simulink model "VCU_CS75_12_30_test"  (R2014a)
settings: Solver=FixedStepDiscrete  StartTime=0.0  StopTime=25  FixedStep=0.0005  RelTol=1e-3
InitFcn:
  | PID_canshu
values from neighbouring files (symbols this model uses):
  D1 = ecucoder_cal(D1)    [PID_canshu.m]
  D2 = ecucoder_cal(D2)    [PID_canshu.m]
  D3 = ecucoder_cal(D3)    [PID_canshu.m]
  ErrorLimit = ecucoder_cal(ErrorLimit)    [PID_canshu.m]
  ErrorSumMax1 = ecucoder_cal(ErrorSumMax1)    [PID_canshu.m]
  ErrorSumMax2 = ecucoder_cal(ErrorSumMax2)    [PID_canshu.m]
  ErrorSumMax3 = ecucoder_cal(ErrorSumMax3)    [PID_canshu.m]
  I1 = ecucoder_cal(I1)    [PID_canshu.m]
  I2 = ecucoder_cal(I2)    [PID_canshu.m]
  I3 = ecucoder_cal(I3)    [PID_canshu.m]
  Limit1 = ecucoder_cal(Limit1)    [PID_canshu.m]
  Limit2 = ecucoder_cal(Limit2)    [PID_canshu.m]
  P1 = ecucoder_cal(P1)    [PID_canshu.m]
  P2 = ecucoder_cal(P2)    [PID_canshu.m]
  P3 = ecucoder_cal(P3)    [PID_canshu.m]
  T_buchang = ecucoder_cal(T_buchang)    [PID_canshu.m]
undefined symbols (not defined in the file or in its folder): ecucoder_acal, I_SW01_L, LaterlAngleCommand, LDW, RemoteAcclPosition
libraries: simulink x940, ec5744lib x41
(part 19 of 31)

== system VCU_CS75_12_30_test/长安CS75底盘程序，20ms一次/Output/Subsystem/2E5/ACC_2E5/ACC_AEBLVehilcehold ==
  ACC_AEBLVehilcehold : Inport
  ACC_AEBLVehilceholdRon : Rounding  Operator=round
  ACC_AEBLVehilcehold_1sat : Saturate  UpperLimit=4  LowerLimit=0
  ACC_AEBLVehilcehold_Convert : DataTypeConversion  OutDataTypeStr=uint8
  ACC_AEBLVehilcehold_Convert1 : DataTypeConversion  OutDataTypeStr=uint32
  ACC_AEBLVehilcehold_D : Product  Inputs=*/
  ACC_AEBLVehilcehold_F : Constant  OutDataTypeStr=single
  ACC_AEBLVehilcehold_L : simulink/Logic and Bit Operations/Bitwise Operator  logicop=AND  UseBitMask=on  BitMask=4  BitMaskRealWorld=Stored Integer
  ACC_AEBLVehilcehold_O : Constant  Value=0  OutDataTypeStr=single
  ACC_AEBLVehilcehold_S : ArithShift  BitShiftNumber=-2
  ACC_AEBLVehilcehold_sat : Saturate  UpperLimit=1  LowerLimit=0
  ACC_AEBLVehilcehold_st : Sum  Inputs=+-
  Constant{1..3,5..8} (7 alike) : Constant  Value=0  OutDataTypeStr=uint8
  output1 : Outport
  output2 : Outport  Port=2
  output3 : Outport  Port=3
  output4 : Outport  Port=4
  output5 : Outport  Port=5
  output6 : Outport  Port=6
  output7 : Outport  Port=7
  output8 : Outport  Port=8
  wires:
  ACC_AEBLVehilcehold/1 -> ACC_AEBLVehilcehold_sat/1
  ACC_AEBLVehilcehold_sat/1 -> ACC_AEBLVehilcehold_st/1
  ACC_AEBLVehilcehold_O/1 -> ACC_AEBLVehilcehold_st/2
  ACC_AEBLVehilcehold_st/1 -> ACC_AEBLVehilcehold_D/1
  ACC_AEBLVehilcehold_F/1 -> ACC_AEBLVehilcehold_D/2
  ACC_AEBLVehilcehold_D/1 -> ACC_AEBLVehilceholdRon/1
  ACC_AEBLVehilceholdRon/1 -> ACC_AEBLVehilcehold_S/1
  ACC_AEBLVehilcehold_S/1 -> ACC_AEBLVehilcehold_1sat/1
  ACC_AEBLVehilcehold_1sat/1 -> ACC_AEBLVehilcehold_Convert1/1
  ACC_AEBLVehilcehold_Convert1/1 -> ACC_AEBLVehilcehold_L/1
  ACC_AEBLVehilcehold_L/1 -> ACC_AEBLVehilcehold_Convert/1
  ACC_AEBLVehilcehold_Convert/1 -> output4/1
  Constant1/1 -> output1/1
  Constant2/1 -> output2/1
  Constant3/1 -> output3/1
  Constant5/1 -> output5/1
  Constant6/1 -> output6/1
  Constant7/1 -> output7/1
  Constant8/1 -> output8/1

== system VCU_CS75_12_30_test/长安CS75底盘程序，20ms一次/Output/Subsystem/2E5/ACC_2E5/ACC_AEBTargetDeceleration ==
  ACC_AEBTargetDeceleration : Inport
  ACC_AEBTargetDecelerationBitCov : DataTypeConversion  OutDataTypeStr=uint32
  ACC_AEBTargetDecelerationBitCov1 : DataTypeConversion  OutDataTypeStr=uint8
  ACC_AEBTargetDecelerationCOV : DataTypeConversion  OutDataTypeStr=uint8
  ACC_AEBTargetDecelerationCOV1 : DataTypeConversion  OutDataTypeStr=uint8
  ACC_AEBTargetDecelerationRon : Rounding  Operator=round
  ACC_AEBTargetDeceleration_1sat : Saturate  UpperLimit=2097120  LowerLimit=0
  ACC_AEBTargetDeceleration_And : simulink/Logic and Bit Operations/Bitwise Operator  logicop=AND  UseBitMask=off  NumInputPorts=2  BitMask=bin2dec('11011001')  BitMaskRealWorld=Stored Integer
  ACC_AEBTargetDeceleration_And1 : simulink/Logic and Bit Operations/Bitwise Operator  logicop=AND  UseBitMask=off  NumInputPorts=2  BitMask=bin2dec('11011001')  BitMaskRealWorld=Stored Integer
  ACC_AEBTargetDeceleration_And1_C : Constant  Value=255  OutDataTypeStr=uint32
  ACC_AEBTargetDeceleration_And_C : Constant  Value=65535
  ACC_AEBTargetDeceleration_Convert : DataTypeConversion  OutDataTypeStr=uint32
  ACC_AEBTargetDeceleration_D : Product  Inputs=*/
  ACC_AEBTargetDeceleration_D1 : Product  Inputs=*/
  ACC_AEBTargetDeceleration_D2 : Product  Inputs=*/
  ACC_AEBTargetDeceleration_F : Constant  Value=0.0005  OutDataTypeStr=single
  ACC_AEBTargetDeceleration_L : simulink/Logic and Bit Operations/Bitwise Operator  logicop=AND  UseBitMask=on  BitMask=2097120  BitMaskRealWorld=Stored Integer
  ACC_AEBTargetDeceleration_O : Constant  Value=-16  OutDataTypeStr=single
  ACC_AEBTargetDeceleration_S : ArithShift  BitShiftNumber=-5
  ACC_AEBTargetDeceleration_sat : Saturate  UpperLimit=16  LowerLimit=-16
  ACC_AEBTargetDeceleration_st : Sum  Inputs=+-
  ACC_AEBTargetDecelerationoutput1_C : Constant  Value=65536
  ACC_AEBTargetDecelerationoutput2_C : Constant  Value=256
  Constant{4..8} (5 alike) : Constant  Value=0  OutDataTypeStr=uint8
  output1 : Outport
  output2 : Outport  Port=2
  output3 : Outport  Port=3
  output4 : Outport  Port=4
  output5 : Outport  Port=5
  output6 : Outport  Port=6
  output7 : Outport  Port=7
  output8 : Outport  Port=8
  wires:
  ACC_AEBTargetDeceleration/1 -> ACC_AEBTargetDeceleration_sat/1
  ACC_AEBTargetDeceleration_sat/1 -> ACC_AEBTargetDeceleration_st/1
  ACC_AEBTargetDeceleration_O/1 -> ACC_AEBTargetDeceleration_st/2
  ACC_AEBTargetDeceleration_st/1 -> ACC_AEBTargetDeceleration_D/1
  ACC_AEBTargetDeceleration_F/1 -> ACC_AEBTargetDeceleration_D/2
  ACC_AEBTargetDeceleration_D/1 -> ACC_AEBTargetDecelerationRon/1
  ACC_AEBTargetDecelerationRon/1 -> ACC_AEBTargetDeceleration_S/1
  ACC_AEBTargetDeceleration_S/1 -> ACC_AEBTargetDeceleration_1sat/1
  ACC_AEBTargetDeceleration_1sat/1 -> ACC_AEBTargetDeceleration_Convert/1
  ACC_AEBTargetDeceleration_Convert/1 -> ACC_AEBTargetDeceleration_L/1
  ACC_AEBTargetDeceleration_L/1 -> ACC_AEBTargetDeceleration_D1/1, ACC_AEBTargetDeceleration_And/1, ACC_AEBTargetDeceleration_And1/1
  ACC_AEBTargetDecelerationoutput1_C/1 -> ACC_AEBTargetDeceleration_D1/2
  ACC_AEBTargetDeceleration_D1/1 -> ACC_AEBTargetDecelerationCOV/1
  ACC_AEBTargetDecelerationCOV/1 -> output1/1
  ACC_AEBTargetDeceleration_And_C/1 -> ACC_AEBTargetDecelerationBitCov/1
  ACC_AEBTargetDecelerationBitCov/1 -> ACC_AEBTargetDeceleration_And/2
  ACC_AEBTargetDeceleration_And/1 -> ACC_AEBTargetDeceleration_D2/1
  ACC_AEBTargetDecelerationoutput2_C/1 -> ACC_AEBTargetDeceleration_D2/2
  ACC_AEBTargetDeceleration_D2/1 -> ACC_AEBTargetDecelerationCOV1/1
  ACC_AEBTargetDecelerationCOV1/1 -> output2/1
  ACC_AEBTargetDeceleration_And1_C/1 -> ACC_AEBTargetDeceleration_And1/2
  ACC_AEBTargetDeceleration_And1/1 -> ACC_AEBTargetDecelerationBitCov1/1
  ACC_AEBTargetDecelerationBitCov1/1 -> output3/1
  Constant4/1 -> output4/1
  Constant5/1 -> output5/1
  Constant6/1 -> output6/1
  Constant7/1 -> output7/1
  Constant8/1 -> output8/1

== system VCU_CS75_12_30_test/长安CS75底盘程序，20ms一次/Output/Subsystem/2E5/ACC_2E5/ACC_AWBavailable ==
  ACC_AWBavailable : Inport
  ACC_AWBavailableRon : Rounding  Operator=round
  ACC_AWBavailable_1sat : Saturate  UpperLimit=128  LowerLimit=0
  ACC_AWBavailable_Convert : DataTypeConversion  OutDataTypeStr=uint8
  ACC_AWBavailable_Convert1 : DataTypeConversion  OutDataTypeStr=uint32
  ACC_AWBavailable_D : Product  Inputs=*/
  ACC_AWBavailable_F : Constant  OutDataTypeStr=single
  ACC_AWBavailable_L : simulink/Logic and Bit Operations/Bitwise Operator  logicop=AND  UseBitMask=on  BitMask=128  BitMaskRealWorld=Stored Integer
  ACC_AWBavailable_O : Constant  Value=0  OutDataTypeStr=single
  ACC_AWBavailable_S : ArithShift  BitShiftNumber=-7
  ACC_AWBavailable_sat : Saturate  UpperLimit=1  LowerLimit=0
  ACC_AWBavailable_st : Sum  Inputs=+-
  Constant{1..3,5..8} (7 alike) : Constant  Value=0  OutDataTypeStr=uint8
  output1 : Outport
  output2 : Outport  Port=2
  output3 : Outport  Port=3
  output4 : Outport  Port=4
  output5 : Outport  Port=5
  output6 : Outport  Port=6
  output7 : Outport  Port=7
  output8 : Outport  Port=8
  wires:
  ACC_AWBavailable/1 -> ACC_AWBavailable_sat/1
  ACC_AWBavailable_sat/1 -> ACC_AWBavailable_st/1
  ACC_AWBavailable_O/1 -> ACC_AWBavailable_st/2
  ACC_AWBavailable_st/1 -> ACC_AWBavailable_D/1
  ACC_AWBavailable_F/1 -> ACC_AWBavailable_D/2
  ACC_AWBavailable_D/1 -> ACC_AWBavailableRon/1
  ACC_AWBavailableRon/1 -> ACC_AWBavailable_S/1
  ACC_AWBavailable_S/1 -> ACC_AWBavailable_1sat/1
  ACC_AWBavailable_1sat/1 -> ACC_AWBavailable_Convert1/1
  ACC_AWBavailable_Convert1/1 -> ACC_AWBavailable_L/1
  ACC_AWBavailable_L/1 -> ACC_AWBavailable_Convert/1
  ACC_AWBavailable_Convert/1 -> output4/1
  Constant1/1 -> output1/1
  Constant2/1 -> output2/1
  Constant3/1 -> output3/1
  Constant5/1 -> output5/1
  Constant6/1 -> output6/1
  Constant7/1 -> output7/1
  Constant8/1 -> output8/1

== system VCU_CS75_12_30_test/长安CS75底盘程序，20ms一次/Output/Subsystem/2E5/ACC_2E5/ACC_AWBlevel ==
  ACC_AWBlevel : Inport
  ACC_AWBlevelRon : Rounding  Operator=round
  ACC_AWBlevel_1sat : Saturate  UpperLimit=15  LowerLimit=0
  ACC_AWBlevel_Convert : DataTypeConversion  OutDataTypeStr=uint8
  ACC_AWBlevel_Convert1 : DataTypeConversion  OutDataTypeStr=uint32
  ACC_AWBlevel_D : Product  Inputs=*/
  ACC_AWBlevel_F : Constant  OutDataTypeStr=single
  ACC_AWBlevel_L : simulink/Logic and Bit Operations/Bitwise Operator  logicop=AND  UseBitMask=on  BitMask=15  BitMaskRealWorld=Stored Integer
  ACC_AWBlevel_O : Constant  Value=0  OutDataTypeStr=single
  ACC_AWBlevel_S : ArithShift
  ACC_AWBlevel_sat : Saturate  UpperLimit=15  LowerLimit=0
  ACC_AWBlevel_st : Sum  Inputs=+-
  Constant{1..2,4..8} (7 alike) : Constant  Value=0  OutDataTypeStr=uint8
  output1 : Outport
  output2 : Outport  Port=2
  output3 : Outport  Port=3
  output4 : Outport  Port=4
  output5 : Outport  Port=5
  output6 : Outport  Port=6
  output7 : Outport  Port=7
  output8 : Outport  Port=8
  wires:
  ACC_AWBlevel/1 -> ACC_AWBlevel_sat/1
  ACC_AWBlevel_sat/1 -> ACC_AWBlevel_st/1
  ACC_AWBlevel_O/1 -> ACC_AWBlevel_st/2
  ACC_AWBlevel_st/1 -> ACC_AWBlevel_D/1
  ACC_AWBlevel_F/1 -> ACC_AWBlevel_D/2
  ACC_AWBlevel_D/1 -> ACC_AWBlevelRon/1
  ACC_AWBlevelRon/1 -> ACC_AWBlevel_S/1
  ACC_AWBlevel_S/1 -> ACC_AWBlevel_1sat/1
  ACC_AWBlevel_1sat/1 -> ACC_AWBlevel_Convert1/1
  ACC_AWBlevel_Convert1/1 -> ACC_AWBlevel_L/1
  ACC_AWBlevel_L/1 -> ACC_AWBlevel_Convert/1
  ACC_AWBlevel_Convert/1 -> output3/1
  Constant1/1 -> output1/1
  Constant2/1 -> output2/1
  Constant4/1 -> output4/1
  Constant5/1 -> output5/1
  Constant6/1 -> output6/1
  Constant7/1 -> output7/1
  Constant8/1 -> output8/1

== system VCU_CS75_12_30_test/长安CS75底盘程序，20ms一次/Output/Subsystem/2E5/ACC_2E5/ACC_AccTorqueReq ==
  ACC_AccTorqueReq : Inport
  ACC_AccTorqueReqBitCov : DataTypeConversion  OutDataTypeStr=uint8
  ACC_AccTorqueReqCOV : DataTypeConversion  OutDataTypeStr=uint8
  ACC_AccTorqueReqRon : Rounding  Operator=round
  ACC_AccTorqueReq_1sat : Saturate  UpperLimit=4092  LowerLimit=0
  ACC_AccTorqueReq_And : simulink/Logic and Bit Operations/Bitwise Operator  logicop=AND  UseBitMask=off  NumInputPorts=2  BitMask=bin2dec('11011001')  BitMaskRealWorld=Stored Integer
  ACC_AccTorqueReq_And_C : Constant  Value=255  OutDataTypeStr=uint32
  ACC_AccTorqueReq_Convert : DataTypeConversion  OutDataTypeStr=uint32
  ACC_AccTorqueReq_D : Product  Inputs=*/
  ACC_AccTorqueReq_D1 : Product  Inputs=*/
  ACC_AccTorqueReq_F : Constant  Value=0.09784  OutDataTypeStr=single
  ACC_AccTorqueReq_L : simulink/Logic and Bit Operations/Bitwise Operator  logicop=AND  UseBitMask=on  BitMask=4092  BitMaskRealWorld=Stored Integer
  ACC_AccTorqueReq_O : Constant  Value=0  OutDataTypeStr=single
  ACC_AccTorqueReq_S : ArithShift  BitShiftNumber=-2
  ACC_AccTorqueReq_sat : Saturate  UpperLimit=100.09032  LowerLimit=0
  ACC_AccTorqueReq_st : Sum  Inputs=+-
  ACC_AccTorqueReqoutput5_C : Constant  Value=256
  Constant{1..4,7..8} (6 alike) : Constant  Value=0  OutDataTypeStr=uint8
  output1 : Outport
  output2 : Outport  Port=2
  output3 : Outport  Port=3
  output4 : Outport  Port=4
  output5 : Outport  Port=5
  output6 : Outport  Port=6
  output7 : Outport  Port=7
  output8 : Outport  Port=8
  wires:
  ACC_AccTorqueReq/1 -> ACC_AccTorqueReq_sat/1
  ACC_AccTorqueReq_sat/1 -> ACC_AccTorqueReq_st/1
  ACC_AccTorqueReq_O/1 -> ACC_AccTorqueReq_st/2
  ACC_AccTorqueReq_st/1 -> ACC_AccTorqueReq_D/1
  ACC_AccTorqueReq_F/1 -> ACC_AccTorqueReq_D/2
  ACC_AccTorqueReq_D/1 -> ACC_AccTorqueReqRon/1
  ACC_AccTorqueReqRon/1 -> ACC_AccTorqueReq_S/1
  ACC_AccTorqueReq_S/1 -> ACC_AccTorqueReq_1sat/1
  ACC_AccTorqueReq_1sat/1 -> ACC_AccTorqueReq_Convert/1
  ACC_AccTorqueReq_Convert/1 -> ACC_AccTorqueReq_L/1
  ACC_AccTorqueReq_L/1 -> ACC_AccTorqueReq_D1/1, ACC_AccTorqueReq_And/1
  ACC_AccTorqueReqoutput5_C/1 -> ACC_AccTorqueReq_D1/2
  ACC_AccTorqueReq_D1/1 -> ACC_AccTorqueReqCOV/1
  ACC_AccTorqueReqCOV/1 -> output5/1
  ACC_AccTorqueReq_And_C/1 -> ACC_AccTorqueReq_And/2
  ACC_AccTorqueReq_And/1 -> ACC_AccTorqueReqBitCov/1
  ACC_AccTorqueReqBitCov/1 -> output6/1
  Constant1/1 -> output1/1
  Constant2/1 -> output2/1
  Constant3/1 -> output3/1
  Constant4/1 -> output4/1
  Constant7/1 -> output7/1
  Constant8/1 -> output8/1

== system VCU_CS75_12_30_test/长安CS75底盘程序，20ms一次/Output/Subsystem/2E5/ACC_2E5/ACC_AccTrqReqEnable ==
  ACC_AccTrqReqEnable : Inport
  ACC_AccTrqReqEnableRon : Rounding  Operator=round
  ACC_AccTrqReqEnable_1sat : Saturate  UpperLimit=128  LowerLimit=0
  ACC_AccTrqReqEnable_Convert : DataTypeConversion  OutDataTypeStr=uint8
  ACC_AccTrqReqEnable_Convert1 : DataTypeConversion  OutDataTypeStr=uint32
  ACC_AccTrqReqEnable_D : Product  Inputs=*/
  ACC_AccTrqReqEnable_F : Constant  OutDataTypeStr=single
  ACC_AccTrqReqEnable_L : simulink/Logic and Bit Operations/Bitwise Operator  logicop=AND  UseBitMask=on  BitMask=128  BitMaskRealWorld=Stored Integer
  ACC_AccTrqReqEnable_O : Constant  Value=0  OutDataTypeStr=single
  ACC_AccTrqReqEnable_S : ArithShift  BitShiftNumber=-7
  ACC_AccTrqReqEnable_sat : Saturate  UpperLimit=1  LowerLimit=0
  ACC_AccTrqReqEnable_st : Sum  Inputs=+-
  Constant{2..8} (7 alike) : Constant  Value=0  OutDataTypeStr=uint8
  output1 : Outport
  output2 : Outport  Port=2
  output3 : Outport  Port=3
  output4 : Outport  Port=4
  output5 : Outport  Port=5
  output6 : Outport  Port=6
  output7 : Outport  Port=7
  output8 : Outport  Port=8
  wires:
  ACC_AccTrqReqEnable/1 -> ACC_AccTrqReqEnable_sat/1
  ACC_AccTrqReqEnable_sat/1 -> ACC_AccTrqReqEnable_st/1
  ACC_AccTrqReqEnable_O/1 -> ACC_AccTrqReqEnable_st/2
  ACC_AccTrqReqEnable_st/1 -> ACC_AccTrqReqEnable_D/1
  ACC_AccTrqReqEnable_F/1 -> ACC_AccTrqReqEnable_D/2
  ACC_AccTrqReqEnable_D/1 -> ACC_AccTrqReqEnableRon/1
  ACC_AccTrqReqEnableRon/1 -> ACC_AccTrqReqEnable_S/1
  ACC_AccTrqReqEnable_S/1 -> ACC_AccTrqReqEnable_1sat/1
  ACC_AccTrqReqEnable_1sat/1 -> ACC_AccTrqReqEnable_Convert1/1
  ACC_AccTrqReqEnable_Convert1/1 -> ACC_AccTrqReqEnable_L/1
  ACC_AccTrqReqEnable_L/1 -> ACC_AccTrqReqEnable_Convert/1
  ACC_AccTrqReqEnable_Convert/1 -> output1/1
  Constant2/1 -> output2/1
  Constant3/1 -> output3/1
  Constant4/1 -> output4/1
  Constant5/1 -> output5/1
  Constant6/1 -> output6/1
  Constant7/1 -> output7/1
  Constant8/1 -> output8/1

== system VCU_CS75_12_30_test/长安CS75底盘程序，20ms一次/Output/Subsystem/2E5/ACC_2E5/ACC_CheckSum ==
  ACC_CheckSum : Inport
  ACC_CheckSumRon : Rounding  Operator=round
  ACC_CheckSum_1sat : Saturate  UpperLimit=255  LowerLimit=0
  ACC_CheckSum_Convert : DataTypeConversion  OutDataTypeStr=uint8
  ACC_CheckSum_Convert1 : DataTypeConversion  OutDataTypeStr=uint32
  ACC_CheckSum_D : Product  Inputs=*/
  ACC_CheckSum_F : Constant  OutDataTypeStr=single
  ACC_CheckSum_L : simulink/Logic and Bit Operations/Bitwise Operator  logicop=AND  UseBitMask=on  BitMask=255  BitMaskRealWorld=Stored Integer
  ACC_CheckSum_O : Constant  Value=0  OutDataTypeStr=single
  ACC_CheckSum_S : ArithShift
  ACC_CheckSum_sat : Saturate  UpperLimit=255  LowerLimit=0
  ACC_CheckSum_st : Sum  Inputs=+-
  Constant{1..7} (7 alike) : Constant  Value=0  OutDataTypeStr=uint8
  output1 : Outport
  output2 : Outport  Port=2
  output3 : Outport  Port=3
  output4 : Outport  Port=4
  output5 : Outport  Port=5
  output6 : Outport  Port=6
  output7 : Outport  Port=7
  output8 : Outport  Port=8
  wires:
  ACC_CheckSum/1 -> ACC_CheckSum_sat/1
  ACC_CheckSum_sat/1 -> ACC_CheckSum_st/1
  ACC_CheckSum_O/1 -> ACC_CheckSum_st/2
  ACC_CheckSum_st/1 -> ACC_CheckSum_D/1
  ACC_CheckSum_F/1 -> ACC_CheckSum_D/2
  ACC_CheckSum_D/1 -> ACC_CheckSumRon/1
  ACC_CheckSumRon/1 -> ACC_CheckSum_S/1
  ACC_CheckSum_S/1 -> ACC_CheckSum_1sat/1
  ACC_CheckSum_1sat/1 -> ACC_CheckSum_Convert1/1
  ACC_CheckSum_Convert1/1 -> ACC_CheckSum_L/1
  ACC_CheckSum_L/1 -> ACC_CheckSum_Convert/1
  ACC_CheckSum_Convert/1 -> output8/1
  Constant1/1 -> output1/1
  Constant2/1 -> output2/1
  Constant3/1 -> output3/1
  Constant4/1 -> output4/1
  Constant5/1 -> output5/1
  Constant6/1 -> output6/1
  Constant7/1 -> output7/1

== system VCU_CS75_12_30_test/长安CS75底盘程序，20ms一次/Output/Subsystem/2E5/ACC_2E5/ACC_ESPPrefill ==
  ACC_ESPPrefill : Inport
  ACC_ESPPrefillRon : Rounding  Operator=round
  ACC_ESPPrefill_1sat : Saturate  UpperLimit=64  LowerLimit=0
  ACC_ESPPrefill_Convert : DataTypeConversion  OutDataTypeStr=uint8
  ACC_ESPPrefill_Convert1 : DataTypeConversion  OutDataTypeStr=uint32
  ACC_ESPPrefill_D : Product  Inputs=*/
  ACC_ESPPrefill_F : Constant  OutDataTypeStr=single
  ACC_ESPPrefill_L : simulink/Logic and Bit Operations/Bitwise Operator  logicop=AND  UseBitMask=on  BitMask=64  BitMaskRealWorld=Stored Integer
  ACC_ESPPrefill_O : Constant  Value=0  OutDataTypeStr=single
  ACC_ESPPrefill_S : ArithShift  BitShiftNumber=-6
  ACC_ESPPrefill_sat : Saturate  UpperLimit=1  LowerLimit=0
  ACC_ESPPrefill_st : Sum  Inputs=+-
  Constant{1..3,5..8} (7 alike) : Constant  Value=0  OutDataTypeStr=uint8
  output1 : Outport
  output2 : Outport  Port=2
  output3 : Outport  Port=3
  output4 : Outport  Port=4
  output5 : Outport  Port=5
  output6 : Outport  Port=6
  output7 : Outport  Port=7
  output8 : Outport  Port=8
  wires:
  ACC_ESPPrefill/1 -> ACC_ESPPrefill_sat/1
  ACC_ESPPrefill_sat/1 -> ACC_ESPPrefill_st/1
  ACC_ESPPrefill_O/1 -> ACC_ESPPrefill_st/2
  ACC_ESPPrefill_st/1 -> ACC_ESPPrefill_D/1
  ACC_ESPPrefill_F/1 -> ACC_ESPPrefill_D/2
  ACC_ESPPrefill_D/1 -> ACC_ESPPrefillRon/1
  ACC_ESPPrefillRon/1 -> ACC_ESPPrefill_S/1
  ACC_ESPPrefill_S/1 -> ACC_ESPPrefill_1sat/1
  ACC_ESPPrefill_1sat/1 -> ACC_ESPPrefill_Convert1/1
  ACC_ESPPrefill_Convert1/1 -> ACC_ESPPrefill_L/1
  ACC_ESPPrefill_L/1 -> ACC_ESPPrefill_Convert/1
  ACC_ESPPrefill_Convert/1 -> output4/1
  Constant1/1 -> output1/1
  Constant2/1 -> output2/1
  Constant3/1 -> output3/1
  Constant5/1 -> output5/1
  Constant6/1 -> output6/1
  Constant7/1 -> output7/1
  Constant8/1 -> output8/1

== system VCU_CS75_12_30_test/长安CS75底盘程序，20ms一次/Output/Subsystem/2E5/ACC_2E5/ACC_PCWPenable ==
  ACC_PCWPenable : Inport
  ACC_PCWPenableRon : Rounding  Operator=round
  ACC_PCWPenable_1sat : Saturate  UpperLimit=32  LowerLimit=0
  ACC_PCWPenable_Convert : DataTypeConversion  OutDataTypeStr=uint8
  ACC_PCWPenable_Convert1 : DataTypeConversion  OutDataTypeStr=uint32
  ACC_PCWPenable_D : Product  Inputs=*/
  ACC_PCWPenable_F : Constant  OutDataTypeStr=single
  ACC_PCWPenable_L : simulink/Logic and Bit Operations/Bitwise Operator  logicop=AND  UseBitMask=on  BitMask=32  BitMaskRealWorld=Stored Integer
  ACC_PCWPenable_O : Constant  Value=0  OutDataTypeStr=single
  ACC_PCWPenable_S : ArithShift  BitShiftNumber=-5
  ACC_PCWPenable_sat : Saturate  UpperLimit=1  LowerLimit=0
  ACC_PCWPenable_st : Sum  Inputs=+-
  Constant{1..3,5..8} (7 alike) : Constant  Value=0  OutDataTypeStr=uint8
  output1 : Outport
  output2 : Outport  Port=2
  output3 : Outport  Port=3
  output4 : Outport  Port=4
  output5 : Outport  Port=5
  output6 : Outport  Port=6
  output7 : Outport  Port=7
  output8 : Outport  Port=8
  wires:
  ACC_PCWPenable/1 -> ACC_PCWPenable_sat/1
  ACC_PCWPenable_sat/1 -> ACC_PCWPenable_st/1
  ACC_PCWPenable_O/1 -> ACC_PCWPenable_st/2
  ACC_PCWPenable_st/1 -> ACC_PCWPenable_D/1
  ACC_PCWPenable_F/1 -> ACC_PCWPenable_D/2
  ACC_PCWPenable_D/1 -> ACC_PCWPenableRon/1
  ACC_PCWPenableRon/1 -> ACC_PCWPenable_S/1
  ACC_PCWPenable_S/1 -> ACC_PCWPenable_1sat/1
  ACC_PCWPenable_1sat/1 -> ACC_PCWPenable_Convert1/1
  ACC_PCWPenable_Convert1/1 -> ACC_PCWPenable_L/1
  ACC_PCWPenable_L/1 -> ACC_PCWPenable_Convert/1
  ACC_PCWPenable_Convert/1 -> output4/1
  Constant1/1 -> output1/1
  Constant2/1 -> output2/1
  Constant3/1 -> output3/1
  Constant5/1 -> output5/1
  Constant6/1 -> output6/1
  Constant7/1 -> output7/1
  Constant8/1 -> output8/1

== system VCU_CS75_12_30_test/长安CS75底盘程序，20ms一次/Output/Subsystem/2E5/ACC_2E5/ACC_PCWPreWarning ==
  ACC_PCWPreWarning : Inport
  ACC_PCWPreWarningRon : Rounding  Operator=round
  ACC_PCWPreWarning_1sat : Saturate  UpperLimit=8  LowerLimit=0
  ACC_PCWPreWarning_Convert : DataTypeConversion  OutDataTypeStr=uint8
  ACC_PCWPreWarning_Convert1 : DataTypeConversion  OutDataTypeStr=uint32
  ACC_PCWPreWarning_D : Product  Inputs=*/
  ACC_PCWPreWarning_F : Constant  OutDataTypeStr=single
  ACC_PCWPreWarning_L : simulink/Logic and Bit Operations/Bitwise Operator  logicop=AND  UseBitMask=on  BitMask=8  BitMaskRealWorld=Stored Integer
  ACC_PCWPreWarning_O : Constant  Value=0  OutDataTypeStr=single
  ACC_PCWPreWarning_S : ArithShift  BitShiftNumber=-3
  ACC_PCWPreWarning_sat : Saturate  UpperLimit=0  LowerLimit=0
  ACC_PCWPreWarning_st : Sum  Inputs=+-
  Constant{1..3,5..8} (7 alike) : Constant  Value=0  OutDataTypeStr=uint8
  output1 : Outport
  output2 : Outport  Port=2
  output3 : Outport  Port=3
  output4 : Outport  Port=4
  output5 : Outport  Port=5
  output6 : Outport  Port=6
  output7 : Outport  Port=7
  output8 : Outport  Port=8
  wires:
  ACC_PCWPreWarning/1 -> ACC_PCWPreWarning_sat/1
  ACC_PCWPreWarning_sat/1 -> ACC_PCWPreWarning_st/1
  ACC_PCWPreWarning_O/1 -> ACC_PCWPreWarning_st/2
  ACC_PCWPreWarning_st/1 -> ACC_PCWPreWarning_D/1
  ACC_PCWPreWarning_F/1 -> ACC_PCWPreWarning_D/2
  ACC_PCWPreWarning_D/1 -> ACC_PCWPreWarningRon/1
  ACC_PCWPreWarningRon/1 -> ACC_PCWPreWarning_S/1
  ACC_PCWPreWarning_S/1 -> ACC_PCWPreWarning_1sat/1
  ACC_PCWPreWarning_1sat/1 -> ACC_PCWPreWarning_Convert1/1
  ACC_PCWPreWarning_Convert1/1 -> ACC_PCWPreWarning_L/1
  ACC_PCWPreWarning_L/1 -> ACC_PCWPreWarning_Convert/1
  ACC_PCWPreWarning_Convert/1 -> output4/1
  Constant1/1 -> output1/1
  Constant2/1 -> output2/1
  Constant3/1 -> output3/1
  Constant5/1 -> output5/1
  Constant6/1 -> output6/1
  Constant7/1 -> output7/1
  Constant8/1 -> output8/1

== system VCU_CS75_12_30_test/长安CS75底盘程序，20ms一次/Output/Subsystem/2E5/ACC_2E5/ACC_PCW_LatentWarning ==
  ACC_PCW_LatentWarning : Inport
  ACC_PCW_LatentWarningRon : Rounding  Operator=round
  ACC_PCW_LatentWarning_1sat : Saturate  UpperLimit=16  LowerLimit=0
  ACC_PCW_LatentWarning_Convert : DataTypeConversion  OutDataTypeStr=uint8
  ACC_PCW_LatentWarning_Convert1 : DataTypeConversion  OutDataTypeStr=uint32
  ACC_PCW_LatentWarning_D : Product  Inputs=*/
  ACC_PCW_LatentWarning_F : Constant  OutDataTypeStr=single
  ACC_PCW_LatentWarning_L : simulink/Logic and Bit Operations/Bitwise Operator  logicop=AND  UseBitMask=on  BitMask=16  BitMaskRealWorld=Stored Integer
  ACC_PCW_LatentWarning_O : Constant  Value=0  OutDataTypeStr=single
  ACC_PCW_LatentWarning_S : ArithShift  BitShiftNumber=-4
  ACC_PCW_LatentWarning_sat : Saturate  UpperLimit=0  LowerLimit=0
  ACC_PCW_LatentWarning_st : Sum  Inputs=+-
  Constant{1..3,5..8} (7 alike) : Constant  Value=0  OutDataTypeStr=uint8
  output1 : Outport
  output2 : Outport  Port=2
  output3 : Outport  Port=3
  output4 : Outport  Port=4
  output5 : Outport  Port=5
  output6 : Outport  Port=6
  output7 : Outport  Port=7
  output8 : Outport  Port=8
  wires:
  ACC_PCW_LatentWarning/1 -> ACC_PCW_LatentWarning_sat/1
  ACC_PCW_LatentWarning_sat/1 -> ACC_PCW_LatentWarning_st/1
  ACC_PCW_LatentWarning_O/1 -> ACC_PCW_LatentWarning_st/2
  ACC_PCW_LatentWarning_st/1 -> ACC_PCW_LatentWarning_D/1
  ACC_PCW_LatentWarning_F/1 -> ACC_PCW_LatentWarning_D/2
  ACC_PCW_LatentWarning_D/1 -> ACC_PCW_LatentWarningRon/1
  ACC_PCW_LatentWarningRon/1 -> ACC_PCW_LatentWarning_S/1
  ACC_PCW_LatentWarning_S/1 -> ACC_PCW_LatentWarning_1sat/1
  ACC_PCW_LatentWarning_1sat/1 -> ACC_PCW_LatentWarning_Convert1/1
  ACC_PCW_LatentWarning_Convert1/1 -> ACC_PCW_LatentWarning_L/1
  ACC_PCW_LatentWarning_L/1 -> ACC_PCW_LatentWarning_Convert/1
  ACC_PCW_LatentWarning_Convert/1 -> output4/1
  Constant1/1 -> output1/1
  Constant2/1 -> output2/1
  Constant3/1 -> output3/1
  Constant5/1 -> output5/1
  Constant6/1 -> output6/1
  Constant7/1 -> output7/1
  Constant8/1 -> output8/1

== system VCU_CS75_12_30_test/长安CS75底盘程序，20ms一次/Output/Subsystem/2E5/ACC_2E5/ACC_RollingCounter ==
  ACC_RollingCounter : Inport
  ACC_RollingCounterRon : Rounding  Operator=round
  ACC_RollingCounter_1sat : Saturate  UpperLimit=15  LowerLimit=0
  ACC_RollingCounter_Convert : DataTypeConversion  OutDataTypeStr=uint8
  ACC_RollingCounter_Convert1 : DataTypeConversion  OutDataTypeStr=uint32
  ACC_RollingCounter_D : Product  Inputs=*/
  ACC_RollingCounter_F : Constant  OutDataTypeStr=single
  ACC_RollingCounter_L : simulink/Logic and Bit Operations/Bitwise Operator  logicop=AND  UseBitMask=on  BitMask=15  BitMaskRealWorld=Stored Integer
  ACC_RollingCounter_O : Constant  Value=0  OutDataTypeStr=single
  ACC_RollingCounter_S : ArithShift
  ACC_RollingCounter_sat : Saturate  UpperLimit=15  LowerLimit=0
  ACC_RollingCounter_st : Sum  Inputs=+-
  Constant{1..6,8} (7 alike) : Constant  Value=0  OutDataTypeStr=uint8
  output1 : Outport
  output2 : Outport  Port=2
  output3 : Outport  Port=3
  output4 : Outport  Port=4
  output5 : Outport  Port=5
  output6 : Outport  Port=6
  output7 : Outport  Port=7
  output8 : Outport  Port=8
  wires:
  ACC_RollingCounter/1 -> ACC_RollingCounter_sat/1
  ACC_RollingCounter_sat/1 -> ACC_RollingCounter_st/1
  ACC_RollingCounter_O/1 -> ACC_RollingCounter_st/2
  ACC_RollingCounter_st/1 -> ACC_RollingCounter_D/1
  ACC_RollingCounter_F/1 -> ACC_RollingCounter_D/2
  ACC_RollingCounter_D/1 -> ACC_RollingCounterRon/1
  ACC_RollingCounterRon/1 -> ACC_RollingCounter_S/1
  ACC_RollingCounter_S/1 -> ACC_RollingCounter_1sat/1
  ACC_RollingCounter_1sat/1 -> ACC_RollingCounter_Convert1/1
  ACC_RollingCounter_Convert1/1 -> ACC_RollingCounter_L/1
  ACC_RollingCounter_L/1 -> ACC_RollingCounter_Convert/1
  ACC_RollingCounter_Convert/1 -> output7/1
  Constant1/1 -> output1/1
  Constant2/1 -> output2/1
  Constant3/1 -> output3/1
  Constant4/1 -> output4/1
  Constant5/1 -> output5/1
  Constant6/1 -> output6/1
  Constant8/1 -> output8/1

== system VCU_CS75_12_30_test/长安CS75底盘程序，20ms一次/Output/Subsystem/2E5/ACC_2E5/ACC_TextInfoForDriver ==
  ACC_TextInfoForDriver : Inport
  ACC_TextInfoForDriverBitCov : DataTypeConversion  OutDataTypeStr=uint8
  ACC_TextInfoForDriverCOV : DataTypeConversion  OutDataTypeStr=uint8
  ACC_TextInfoForDriverRon : Rounding  Operator=round
  ACC_TextInfoForDriver_1sat : Saturate  UpperLimit=992  LowerLimit=0
  ACC_TextInfoForDriver_And : simulink/Logic and Bit Operations/Bitwise Operator  logicop=AND  UseBitMask=off  NumInputPorts=2  BitMask=bin2dec('11011001')  BitMaskRealWorld=Stored Integer
  ACC_TextInfoForDriver_And_C : Constant  Value=255  OutDataTypeStr=uint32
  ACC_TextInfoForDriver_Convert : DataTypeConversion  OutDataTypeStr=uint32
  ACC_TextInfoForDriver_D : Product  Inputs=*/
  ACC_TextInfoForDriver_D1 : Product  Inputs=*/
  ACC_TextInfoForDriver_F : Constant  OutDataTypeStr=single
  ACC_TextInfoForDriver_L : simulink/Logic and Bit Operations/Bitwise Operator  logicop=AND  UseBitMask=on  BitMask=992  BitMaskRealWorld=Stored Integer
  ACC_TextInfoForDriver_O : Constant  Value=0  OutDataTypeStr=single
  ACC_TextInfoForDriver_S : ArithShift  BitShiftNumber=-5
  ACC_TextInfoForDriver_sat : Saturate  UpperLimit=31  LowerLimit=0
  ACC_TextInfoForDriver_st : Sum  Inputs=+-
  ACC_TextInfoForDriveroutput6_C : Constant  Value=256
  Constant{1..5,8} (6 alike) : Constant  Value=0  OutDataTypeStr=uint8
  output1 : Outport
  output2 : Outport  Port=2
  output3 : Outport  Port=3
  output4 : Outport  Port=4
  output5 : Outport  Port=5
  output6 : Outport  Port=6
  output7 : Outport  Port=7
  output8 : Outport  Port=8
  wires:
  ACC_TextInfoForDriver/1 -> ACC_TextInfoForDriver_sat/1
  ACC_TextInfoForDriver_sat/1 -> ACC_TextInfoForDriver_st/1
  ACC_TextInfoForDriver_O/1 -> ACC_TextInfoForDriver_st/2
  ACC_TextInfoForDriver_st/1 -> ACC_TextInfoForDriver_D/1
  ACC_TextInfoForDriver_F/1 -> ACC_TextInfoForDriver_D/2
  ACC_TextInfoForDriver_D/1 -> ACC_TextInfoForDriverRon/1
  ACC_TextInfoForDriverRon/1 -> ACC_TextInfoForDriver_S/1
  ACC_TextInfoForDriver_S/1 -> ACC_TextInfoForDriver_1sat/1
  ACC_TextInfoForDriver_1sat/1 -> ACC_TextInfoForDriver_Convert/1
  ACC_TextInfoForDriver_Convert/1 -> ACC_TextInfoForDriver_L/1
  ACC_TextInfoForDriver_L/1 -> ACC_TextInfoForDriver_D1/1, ACC_TextInfoForDriver_And/1
  ACC_TextInfoForDriveroutput6_C/1 -> ACC_TextInfoForDriver_D1/2
  ACC_TextInfoForDriver_D1/1 -> ACC_TextInfoForDriverCOV/1
  ACC_TextInfoForDriverCOV/1 -> output6/1
  ACC_TextInfoForDriver_And_C/1 -> ACC_TextInfoForDriver_And/2
  ACC_TextInfoForDriver_And/1 -> ACC_TextInfoForDriverBitCov/1
  ACC_TextInfoForDriverBitCov/1 -> output7/1
  Constant1/1 -> output1/1
  Constant2/1 -> output2/1
  Constant3/1 -> output3/1
  Constant4/1 -> output4/1
  Constant5/1 -> output5/1
  Constant8/1 -> output8/1

== system VCU_CS75_12_30_test/长安CS75底盘程序，20ms一次/Output/Subsystem/TransmitMessages1/ACC_34E/ACC_LLaneDistanceFusion ==
  ACC_LLaneDistanceFusion : Inport
  ACC_LLaneDistanceFusionBitCov : DataTypeConversion  OutDataTypeStr=uint8
  ACC_LLaneDistanceFusionCOV : DataTypeConversion  OutDataTypeStr=uint8
  ACC_LLaneDistanceFusionRon : Rounding  Operator=round
  ACC_LLaneDistanceFusion_1sat : Saturate  UpperLimit=2032  LowerLimit=0
  ACC_LLaneDistanceFusion_And : simulink/Logic and Bit Operations/Bitwise Operator  logicop=AND  UseBitMask=off  NumInputPorts=2  BitMask=bin2dec('11011001')  BitMaskRealWorld=Stored Integer
  ACC_LLaneDistanceFusion_And_C : Constant  Value=255  OutDataTypeStr=uint32
  ACC_LLaneDistanceFusion_Convert : DataTypeConversion  OutDataTypeStr=uint32
  ACC_LLaneDistanceFusion_D : Product  Inputs=*/
  ACC_LLaneDistanceFusion_D1 : Product  Inputs=*/
  ACC_LLaneDistanceFusion_F : Constant  Value=0.05  OutDataTypeStr=single
  ACC_LLaneDistanceFusion_L : simulink/Logic and Bit Operations/Bitwise Operator  logicop=AND  UseBitMask=on  BitMask=2032  BitMaskRealWorld=Stored Integer
  ACC_LLaneDistanceFusion_O : Constant  Value=0  OutDataTypeStr=single
  ACC_LLaneDistanceFusion_S : ArithShift  BitShiftNumber=-4
  ACC_LLaneDistanceFusion_sat : Saturate  UpperLimit=6.35  LowerLimit=0
  ACC_LLaneDistanceFusion_st : Sum  Inputs=+-
  ACC_LLaneDistanceFusionoutput3_C : Constant  Value=256
  Constant{1..2,5..8} (6 alike) : Constant  Value=0  OutDataTypeStr=uint8
  output1 : Outport
  output2 : Outport  Port=2
  output3 : Outport  Port=3
  output4 : Outport  Port=4
  output5 : Outport  Port=5
  output6 : Outport  Port=6
  output7 : Outport  Port=7
  output8 : Outport  Port=8
  wires:
  ACC_LLaneDistanceFusion/1 -> ACC_LLaneDistanceFusion_sat/1
  ACC_LLaneDistanceFusion_sat/1 -> ACC_LLaneDistanceFusion_st/1
  ACC_LLaneDistanceFusion_O/1 -> ACC_LLaneDistanceFusion_st/2
  ACC_LLaneDistanceFusion_st/1 -> ACC_LLaneDistanceFusion_D/1
  ACC_LLaneDistanceFusion_F/1 -> ACC_LLaneDistanceFusion_D/2
  ACC_LLaneDistanceFusion_D/1 -> ACC_LLaneDistanceFusionRon/1
  ACC_LLaneDistanceFusionRon/1 -> ACC_LLaneDistanceFusion_S/1
  ACC_LLaneDistanceFusion_S/1 -> ACC_LLaneDistanceFusion_1sat/1
  ACC_LLaneDistanceFusion_1sat/1 -> ACC_LLaneDistanceFusion_Convert/1
  ACC_LLaneDistanceFusion_Convert/1 -> ACC_LLaneDistanceFusion_L/1
  ACC_LLaneDistanceFusion_L/1 -> ACC_LLaneDistanceFusion_D1/1, ACC_LLaneDistanceFusion_And/1
  ACC_LLaneDistanceFusionoutput3_C/1 -> ACC_LLaneDistanceFusion_D1/2
  ACC_LLaneDistanceFusion_D1/1 -> ACC_LLaneDistanceFusionCOV/1
  ACC_LLaneDistanceFusionCOV/1 -> output3/1
  ACC_LLaneDistanceFusion_And_C/1 -> ACC_LLaneDistanceFusion_And/2
  ACC_LLaneDistanceFusion_And/1 -> ACC_LLaneDistanceFusionBitCov/1
  ACC_LLaneDistanceFusionBitCov/1 -> output4/1
  Constant1/1 -> output1/1
  Constant2/1 -> output2/1
  Constant5/1 -> output5/1
  Constant6/1 -> output6/1
  Constant7/1 -> output7/1
  Constant8/1 -> output8/1

== system VCU_CS75_12_30_test/长安CS75底盘程序，20ms一次/Output/Subsystem/TransmitMessages1/ACC_34E/ACC_LeftTargetID ==
  ACC_LeftTargetID : Inport
  ACC_LeftTargetIDRon : Rounding  Operator=round
  ACC_LeftTargetID_1sat : Saturate  UpperLimit=15  LowerLimit=0
  ACC_LeftTargetID_Convert : DataTypeConversion  OutDataTypeStr=uint8
  ACC_LeftTargetID_Convert1 : DataTypeConversion  OutDataTypeStr=uint32
  ACC_LeftTargetID_D : Product  Inputs=*/
  ACC_LeftTargetID_F : Constant  OutDataTypeStr=single
  ACC_LeftTargetID_L : simulink/Logic and Bit Operations/Bitwise Operator  logicop=AND  UseBitMask=on  BitMask=15  BitMaskRealWorld=Stored Integer
  ACC_LeftTargetID_O : Constant  Value=0  OutDataTypeStr=single
  ACC_LeftTargetID_S : ArithShift
  ACC_LeftTargetID_sat : Saturate  UpperLimit=15  LowerLimit=0
  ACC_LeftTargetID_st : Sum  Inputs=+-
  Constant{2..8} (7 alike) : Constant  Value=0  OutDataTypeStr=uint8
  output1 : Outport
  output2 : Outport  Port=2
  output3 : Outport  Port=3
  output4 : Outport  Port=4
  output5 : Outport  Port=5
  output6 : Outport  Port=6
  output7 : Outport  Port=7
  output8 : Outport  Port=8
  wires:
  ACC_LeftTargetID/1 -> ACC_LeftTargetID_sat/1
  ACC_LeftTargetID_sat/1 -> ACC_LeftTargetID_st/1
  ACC_LeftTargetID_O/1 -> ACC_LeftTargetID_st/2
  ACC_LeftTargetID_st/1 -> ACC_LeftTargetID_D/1
  ACC_LeftTargetID_F/1 -> ACC_LeftTargetID_D/2
  ACC_LeftTargetID_D/1 -> ACC_LeftTargetIDRon/1
  ACC_LeftTargetIDRon/1 -> ACC_LeftTargetID_S/1
  ACC_LeftTargetID_S/1 -> ACC_LeftTargetID_1sat/1
  ACC_LeftTargetID_1sat/1 -> ACC_LeftTargetID_Convert1/1
  ACC_LeftTargetID_Convert1/1 -> ACC_LeftTargetID_L/1
  ACC_LeftTargetID_L/1 -> ACC_LeftTargetID_Convert/1
  ACC_LeftTargetID_Convert/1 -> output1/1
  Constant2/1 -> output2/1
  Constant3/1 -> output3/1
  Constant4/1 -> output4/1
  Constant5/1 -> output5/1
  Constant6/1 -> output6/1
  Constant7/1 -> output7/1
  Constant8/1 -> output8/1

== system VCU_CS75_12_30_test/长安CS75底盘程序，20ms一次/Output/Subsystem/TransmitMessages1/ACC_34E/ACC_RLaneDistanceFusion ==
  ACC_RLaneDistanceFusion : Inport
  ACC_RLaneDistanceFusionBitCov : DataTypeConversion  OutDataTypeStr=uint8
  ACC_RLaneDistanceFusionCOV : DataTypeConversion  OutDataTypeStr=uint8
  ACC_RLaneDistanceFusionRon : Rounding  Operator=round
  ACC_RLaneDistanceFusion_1sat : Saturate  UpperLimit=1016  LowerLimit=0
  ACC_RLaneDistanceFusion_And : simulink/Logic and Bit Operations/Bitwise Operator  logicop=AND  UseBitMask=off  NumInputPorts=2  BitMask=bin2dec('11011001')  BitMaskRealWorld=Stored Integer
  ACC_RLaneDistanceFusion_And_C : Constant  Value=255  OutDataTypeStr=uint32
  ACC_RLaneDistanceFusion_Convert : DataTypeConversion  OutDataTypeStr=uint32
  ACC_RLaneDistanceFusion_D : Product  Inputs=*/
  ACC_RLaneDistanceFusion_D1 : Product  Inputs=*/
  ACC_RLaneDistanceFusion_F : Constant  Value=0.05  OutDataTypeStr=single
  ACC_RLaneDistanceFusion_L : simulink/Logic and Bit Operations/Bitwise Operator  logicop=AND  UseBitMask=on  BitMask=1016  BitMaskRealWorld=Stored Integer
  ACC_RLaneDistanceFusion_O : Constant  Value=0  OutDataTypeStr=single
  ACC_RLaneDistanceFusion_S : ArithShift  BitShiftNumber=-3
  ACC_RLaneDistanceFusion_sat : Saturate  UpperLimit=6.35  LowerLimit=0
  ACC_RLaneDistanceFusion_st : Sum  Inputs=+-
  ACC_RLaneDistanceFusionoutput2_C : Constant  Value=256
  Constant{1,4..8} (6 alike) : Constant  Value=0  OutDataTypeStr=uint8
  output1 : Outport
  output2 : Outport  Port=2
  output3 : Outport  Port=3
  output4 : Outport  Port=4
  output5 : Outport  Port=5
  output6 : Outport  Port=6
  output7 : Outport  Port=7
  output8 : Outport  Port=8
  wires:
  ACC_RLaneDistanceFusion/1 -> ACC_RLaneDistanceFusion_sat/1
  ACC_RLaneDistanceFusion_sat/1 -> ACC_RLaneDistanceFusion_st/1
  ACC_RLaneDistanceFusion_O/1 -> ACC_RLaneDistanceFusion_st/2
  ACC_RLaneDistanceFusion_st/1 -> ACC_RLaneDistanceFusion_D/1
  ACC_RLaneDistanceFusion_F/1 -> ACC_RLaneDistanceFusion_D/2
  ACC_RLaneDistanceFusion_D/1 -> ACC_RLaneDistanceFusionRon/1
  ACC_RLaneDistanceFusionRon/1 -> ACC_RLaneDistanceFusion_S/1
  ACC_RLaneDistanceFusion_S/1 -> ACC_RLaneDistanceFusion_1sat/1
  ACC_RLaneDistanceFusion_1sat/1 -> ACC_RLaneDistanceFusion_Convert/1
  ACC_RLaneDistanceFusion_Convert/1 -> ACC_RLaneDistanceFusion_L/1
  ACC_RLaneDistanceFusion_L/1 -> ACC_RLaneDistanceFusion_D1/1, ACC_RLaneDistanceFusion_And/1
  ACC_RLaneDistanceFusionoutput2_C/1 -> ACC_RLaneDistanceFusion_D1/2
  ACC_RLaneDistanceFusion_D1/1 -> ACC_RLaneDistanceFusionCOV/1
  ACC_RLaneDistanceFusionCOV/1 -> output2/1
  ACC_RLaneDistanceFusion_And_C/1 -> ACC_RLaneDistanceFusion_And/2
  ACC_RLaneDistanceFusion_And/1 -> ACC_RLaneDistanceFusionBitCov/1
  ACC_RLaneDistanceFusionBitCov/1 -> output3/1
  Constant1/1 -> output1/1
  Constant4/1 -> output4/1
  Constant5/1 -> output5/1
  Constant6/1 -> output6/1
  Constant7/1 -> output7/1
  Constant8/1 -> output8/1

== system VCU_CS75_12_30_test/长安CS75底盘程序，20ms一次/Output/Subsystem/TransmitMessages1/ACC_34E/ACC_RelevantTargetDection ==
  ACC_RelevantTargetDection : Inport
  ACC_RelevantTargetDectionRon : Rounding  Operator=round
  ACC_RelevantTargetDection_1sat : Saturate  UpperLimit=12  LowerLimit=0
  ACC_RelevantTargetDection_Convert : DataTypeConversion  OutDataTypeStr=uint8
  ACC_RelevantTargetDection_Convert1 : DataTypeConversion  OutDataTypeStr=uint32
  ACC_RelevantTargetDection_D : Product  Inputs=*/
  ACC_RelevantTargetDection_F : Constant  OutDataTypeStr=single
  ACC_RelevantTargetDection_L : simulink/Logic and Bit Operations/Bitwise Operator  logicop=AND  UseBitMask=on  BitMask=12  BitMaskRealWorld=Stored Integer
  ACC_RelevantTargetDection_O : Constant  Value=0  OutDataTypeStr=single
  ACC_RelevantTargetDection_S : ArithShift  BitShiftNumber=-2
  ACC_RelevantTargetDection_sat : Saturate  UpperLimit=3  LowerLimit=0
  ACC_RelevantTargetDection_st : Sum  Inputs=+-
  Constant{1,3..8} (7 alike) : Constant  Value=0  OutDataTypeStr=uint8
  output1 : Outport
  output2 : Outport  Port=2
  output3 : Outport  Port=3
  output4 : Outport  Port=4
  output5 : Outport  Port=5
  output6 : Outport  Port=6
  output7 : Outport  Port=7
  output8 : Outport  Port=8
  wires:
  ACC_RelevantTargetDection/1 -> ACC_RelevantTargetDection_sat/1
  ACC_RelevantTargetDection_sat/1 -> ACC_RelevantTargetDection_st/1
  ACC_RelevantTargetDection_O/1 -> ACC_RelevantTargetDection_st/2
  ACC_RelevantTargetDection_st/1 -> ACC_RelevantTargetDection_D/1
  ACC_RelevantTargetDection_F/1 -> ACC_RelevantTargetDection_D/2
  ACC_RelevantTargetDection_D/1 -> ACC_RelevantTargetDectionRon/1
  ACC_RelevantTargetDectionRon/1 -> ACC_RelevantTargetDection_S/1
  ACC_RelevantTargetDection_S/1 -> ACC_RelevantTargetDection_1sat/1
  ACC_RelevantTargetDection_1sat/1 -> ACC_RelevantTargetDection_Convert1/1
  ACC_RelevantTargetDection_Convert1/1 -> ACC_RelevantTargetDection_L/1
  ACC_RelevantTargetDection_L/1 -> ACC_RelevantTargetDection_Convert/1
  ACC_RelevantTargetDection_Convert/1 -> output2/1
  Constant1/1 -> output1/1
  Constant3/1 -> output3/1
  Constant4/1 -> output4/1
  Constant5/1 -> output5/1
  Constant6/1 -> output6/1
  Constant7/1 -> output7/1
  Constant8/1 -> output8/1

== system VCU_CS75_12_30_test/长安CS75底盘程序，20ms一次/Output/Subsystem/TransmitMessages1/ACC_34E/ACC_RelevantTargetID ==
  ACC_RelevantTargetID : Inport
  ACC_RelevantTargetIDRon : Rounding  Operator=round
  ACC_RelevantTargetID_1sat : Saturate  UpperLimit=240  LowerLimit=0
  ACC_RelevantTargetID_Convert : DataTypeConversion  OutDataTypeStr=uint8
  ACC_RelevantTargetID_Convert1 : DataTypeConversion  OutDataTypeStr=uint32
  ACC_RelevantTargetID_D : Product  Inputs=*/
  ACC_RelevantTargetID_F : Constant  OutDataTypeStr=single
  ACC_RelevantTargetID_L : simulink/Logic and Bit Operations/Bitwise Operator  logicop=AND  UseBitMask=on  BitMask=240  BitMaskRealWorld=Stored Integer
  ACC_RelevantTargetID_O : Constant  Value=0  OutDataTypeStr=single
  ACC_RelevantTargetID_S : ArithShift  BitShiftNumber=-4
  ACC_RelevantTargetID_sat : Saturate  UpperLimit=15  LowerLimit=0
  ACC_RelevantTargetID_st : Sum  Inputs=+-
  Constant{2..8} (7 alike) : Constant  Value=0  OutDataTypeStr=uint8
  output1 : Outport
  output2 : Outport  Port=2
  output3 : Outport  Port=3
  output4 : Outport  Port=4
  output5 : Outport  Port=5
  output6 : Outport  Port=6
  output7 : Outport  Port=7
  output8 : Outport  Port=8
  wires:
  ACC_RelevantTargetID/1 -> ACC_RelevantTargetID_sat/1
  ACC_RelevantTargetID_sat/1 -> ACC_RelevantTargetID_st/1
  ACC_RelevantTargetID_O/1 -> ACC_RelevantTargetID_st/2
  ACC_RelevantTargetID_st/1 -> ACC_RelevantTargetID_D/1
  ACC_RelevantTargetID_F/1 -> ACC_RelevantTargetID_D/2
  ACC_RelevantTargetID_D/1 -> ACC_RelevantTargetIDRon/1
  ACC_RelevantTargetIDRon/1 -> ACC_RelevantTargetID_S/1
  ACC_RelevantTargetID_S/1 -> ACC_RelevantTargetID_1sat/1
  ACC_RelevantTargetID_1sat/1 -> ACC_RelevantTargetID_Convert1/1
  ACC_RelevantTargetID_Convert1/1 -> ACC_RelevantTargetID_L/1
  ACC_RelevantTargetID_L/1 -> ACC_RelevantTargetID_Convert/1
  ACC_RelevantTargetID_Convert/1 -> output1/1
  Constant2/1 -> output2/1
  Constant3/1 -> output3/1
  Constant4/1 -> output4/1
  Constant5/1 -> output5/1
  Constant6/1 -> output6/1
  Constant7/1 -> output7/1
  Constant8/1 -> output8/1

== system VCU_CS75_12_30_test/长安CS75底盘程序，20ms一次/Output/Subsystem/TransmitMessages1/ACC_34E/ACC_RightTargetID ==
  ACC_RightTargetID : Inport
  ACC_RightTargetIDRon : Rounding  Operator=round
  ACC_RightTargetID_1sat : Saturate  UpperLimit=240  LowerLimit=0
  ACC_RightTargetID_Convert : DataTypeConversion  OutDataTypeStr=uint8
  ACC_RightTargetID_Convert1 : DataTypeConversion  OutDataTypeStr=uint32
  ACC_RightTargetID_D : Product  Inputs=*/
  ACC_RightTargetID_F : Constant  OutDataTypeStr=single
  ACC_RightTargetID_L : simulink/Logic and Bit Operations/Bitwise Operator  logicop=AND  UseBitMask=on  BitMask=240  BitMaskRealWorld=Stored Integer
  ACC_RightTargetID_O : Constant  Value=0  OutDataTypeStr=single
  ACC_RightTargetID_S : ArithShift  BitShiftNumber=-4
  ACC_RightTargetID_sat : Saturate  UpperLimit=15  LowerLimit=0
  ACC_RightTargetID_st : Sum  Inputs=+-
  Constant{1,3..8} (7 alike) : Constant  Value=0  OutDataTypeStr=uint8
  output1 : Outport
  output2 : Outport  Port=2
  output3 : Outport  Port=3
  output4 : Outport  Port=4
  output5 : Outport  Port=5
  output6 : Outport  Port=6
  output7 : Outport  Port=7
  output8 : Outport  Port=8
  wires:
  ACC_RightTargetID/1 -> ACC_RightTargetID_sat/1
  ACC_RightTargetID_sat/1 -> ACC_RightTargetID_st/1
  ACC_RightTargetID_O/1 -> ACC_RightTargetID_st/2
  ACC_RightTargetID_st/1 -> ACC_RightTargetID_D/1
  ACC_RightTargetID_F/1 -> ACC_RightTargetID_D/2
  ACC_RightTargetID_D/1 -> ACC_RightTargetIDRon/1
  ACC_RightTargetIDRon/1 -> ACC_RightTargetID_S/1
  ACC_RightTargetID_S/1 -> ACC_RightTargetID_1sat/1
  ACC_RightTargetID_1sat/1 -> ACC_RightTargetID_Convert1/1
  ACC_RightTargetID_Convert1/1 -> ACC_RightTargetID_L/1
  ACC_RightTargetID_L/1 -> ACC_RightTargetID_Convert/1
  ACC_RightTargetID_Convert/1 -> output2/1
  Constant1/1 -> output1/1
  Constant3/1 -> output3/1
  Constant4/1 -> output4/1
  Constant5/1 -> output5/1
  Constant6/1 -> output6/1
  Constant7/1 -> output7/1
  Constant8/1 -> output8/1

== system VCU_CS75_12_30_test/长安CS75底盘程序，20ms一次/Output/Subsystem/TransmitMessages10/LAS_29D/CRC ==
  CRC : Inport
  CRCRon : Rounding  Operator=round
  CRC_1sat : Saturate  UpperLimit=255  LowerLimit=0
  CRC_Convert : DataTypeConversion  OutDataTypeStr=uint8
  CRC_Convert1 : DataTypeConversion  OutDataTypeStr=uint32
  CRC_D : Product  Inputs=*/
  CRC_F : Constant  OutDataTypeStr=single
  CRC_L : simulink/Logic and Bit Operations/Bitwise Operator  logicop=AND  UseBitMask=on  BitMask=255  BitMaskRealWorld=Stored Integer
  CRC_O : Constant  Value=0  OutDataTypeStr=single
  CRC_S : ArithShift
  CRC_sat : Saturate  UpperLimit=0  LowerLimit=0
  CRC_st : Sum  Inputs=+-
  Constant{1..7} (7 alike) : Constant  Value=0  OutDataTypeStr=uint8
  output1 : Outport
  output2 : Outport  Port=2
  output3 : Outport  Port=3
  output4 : Outport  Port=4
  output5 : Outport  Port=5
  output6 : Outport  Port=6
  output7 : Outport  Port=7
  output8 : Outport  Port=8
  wires:
  CRC/1 -> CRC_sat/1
  CRC_sat/1 -> CRC_st/1
  CRC_O/1 -> CRC_st/2
  CRC_st/1 -> CRC_D/1
  CRC_F/1 -> CRC_D/2
  CRC_D/1 -> CRCRon/1
  CRCRon/1 -> CRC_S/1
  CRC_S/1 -> CRC_1sat/1
  CRC_1sat/1 -> CRC_Convert1/1
  CRC_Convert1/1 -> CRC_L/1
  CRC_L/1 -> CRC_Convert/1
  CRC_Convert/1 -> output8/1
  Constant1/1 -> output1/1
  Constant2/1 -> output2/1
  Constant3/1 -> output3/1
  Constant4/1 -> output4/1
  Constant5/1 -> output5/1
  Constant6/1 -> output6/1
  Constant7/1 -> output7/1

== system VCU_CS75_12_30_test/长安CS75底盘程序，20ms一次/Output/Subsystem/TransmitMessages10/LAS_29D/LAS_FatigueDectionEnableStatus ==
  LAS_FatigueDectionEnableStatus : Inport
  Constant{1,3..8} (7 alike) : Constant  Value=0  OutDataTypeStr=uint8
  LAS_FatigueDectionEnableStatusRon : Rounding  Operator=round
  LAS_FatigueDectionEnableStatus_1sat : Saturate  UpperLimit=12  LowerLimit=0
  LAS_FatigueDectionEnableStatus_Convert : DataTypeConversion  OutDataTypeStr=uint8
  LAS_FatigueDectionEnableStatus_Convert1 : DataTypeConversion  OutDataTypeStr=uint32
  LAS_FatigueDectionEnableStatus_D : Product  Inputs=*/
  LAS_FatigueDectionEnableStatus_F : Constant  OutDataTypeStr=single
  LAS_FatigueDectionEnableStatus_L : simulink/Logic and Bit Operations/Bitwise Operator  logicop=AND  UseBitMask=on  BitMask=12  BitMaskRealWorld=Stored Integer
  LAS_FatigueDectionEnableStatus_O : Constant  Value=0  OutDataTypeStr=single
  LAS_FatigueDectionEnableStatus_S : ArithShift  BitShiftNumber=-2
  LAS_FatigueDectionEnableStatus_sat : Saturate  UpperLimit=3  LowerLimit=0
  LAS_FatigueDectionEnableStatus_st : Sum  Inputs=+-
  output1 : Outport
  output2 : Outport  Port=2
  output3 : Outport  Port=3
  output4 : Outport  Port=4
  output5 : Outport  Port=5
  output6 : Outport  Port=6
  output7 : Outport  Port=7
  output8 : Outport  Port=8
  wires:
  LAS_FatigueDectionEnableStatus/1 -> LAS_FatigueDectionEnableStatus_sat/1
  LAS_FatigueDectionEnableStatus_sat/1 -> LAS_FatigueDectionEnableStatus_st/1
  LAS_FatigueDectionEnableStatus_O/1 -> LAS_FatigueDectionEnableStatus_st/2
  LAS_FatigueDectionEnableStatus_st/1 -> LAS_FatigueDectionEnableStatus_D/1
  LAS_FatigueDectionEnableStatus_F/1 -> LAS_FatigueDectionEnableStatus_D/2
  LAS_FatigueDectionEnableStatus_D/1 -> LAS_FatigueDectionEnableStatusRon/1
  LAS_FatigueDectionEnableStatusRon/1 -> LAS_FatigueDectionEnableStatus_S/1
  LAS_FatigueDectionEnableStatus_S/1 -> LAS_FatigueDectionEnableStatus_1sat/1
  LAS_FatigueDectionEnableStatus_1sat/1 -> LAS_FatigueDectionEnableStatus_Convert1/1
  LAS_FatigueDectionEnableStatus_Convert1/1 -> LAS_FatigueDectionEnableStatus_L/1
  LAS_FatigueDectionEnableStatus_L/1 -> LAS_FatigueDectionEnableStatus_Convert/1
  LAS_FatigueDectionEnableStatus_Convert/1 -> output2/1
  Constant1/1 -> output1/1
  Constant3/1 -> output3/1
  Constant4/1 -> output4/1
  Constant5/1 -> output5/1
  Constant6/1 -> output6/1
  Constant7/1 -> output7/1
  Constant8/1 -> output8/1

== system VCU_CS75_12_30_test/长安CS75底盘程序，20ms一次/Output/Subsystem/TransmitMessages10/LAS_29D/LAS_HMAEnableStatus ==
  LAS_HMAEnableStatus : Inport
  Constant{2..8} (7 alike) : Constant  Value=0  OutDataTypeStr=uint8
  LAS_HMAEnableStatusRon : Rounding  Operator=round
  LAS_HMAEnableStatus_1sat : Saturate  UpperLimit=4  LowerLimit=0
  LAS_HMAEnableStatus_Convert : DataTypeConversion  OutDataTypeStr=uint8
  LAS_HMAEnableStatus_Convert1 : DataTypeConversion  OutDataTypeStr=uint32
  LAS_HMAEnableStatus_D : Product  Inputs=*/
  LAS_HMAEnableStatus_F : Constant  OutDataTypeStr=single
  LAS_HMAEnableStatus_L : simulink/Logic and Bit Operations/Bitwise Operator  logicop=AND  UseBitMask=on  BitMask=4  BitMaskRealWorld=Stored Integer
  LAS_HMAEnableStatus_O : Constant  Value=0  OutDataTypeStr=single
  LAS_HMAEnableStatus_S : ArithShift  BitShiftNumber=-2
  LAS_HMAEnableStatus_sat : Saturate  UpperLimit=1  LowerLimit=0
  LAS_HMAEnableStatus_st : Sum  Inputs=+-
  output1 : Outport
  output2 : Outport  Port=2
  output3 : Outport  Port=3
  output4 : Outport  Port=4
  output5 : Outport  Port=5
  output6 : Outport  Port=6
  output7 : Outport  Port=7
  output8 : Outport  Port=8
  wires:
  LAS_HMAEnableStatus/1 -> LAS_HMAEnableStatus_sat/1
  LAS_HMAEnableStatus_sat/1 -> LAS_HMAEnableStatus_st/1
  LAS_HMAEnableStatus_O/1 -> LAS_HMAEnableStatus_st/2
  LAS_HMAEnableStatus_st/1 -> LAS_HMAEnableStatus_D/1
  LAS_HMAEnableStatus_F/1 -> LAS_HMAEnableStatus_D/2
  LAS_HMAEnableStatus_D/1 -> LAS_HMAEnableStatusRon/1
  LAS_HMAEnableStatusRon/1 -> LAS_HMAEnableStatus_S/1
  LAS_HMAEnableStatus_S/1 -> LAS_HMAEnableStatus_1sat/1
  LAS_HMAEnableStatus_1sat/1 -> LAS_HMAEnableStatus_Convert1/1
  LAS_HMAEnableStatus_Convert1/1 -> LAS_HMAEnableStatus_L/1
  LAS_HMAEnableStatus_L/1 -> LAS_HMAEnableStatus_Convert/1
  LAS_HMAEnableStatus_Convert/1 -> output1/1
  Constant2/1 -> output2/1
  Constant3/1 -> output3/1
  Constant4/1 -> output4/1
  Constant5/1 -> output5/1
  Constant6/1 -> output6/1
  Constant7/1 -> output7/1
  Constant8/1 -> output8/1
